simulink model "one_sec_delay_motor_geral_cc"  (R2018b)
settings: Solver=VariableStepAuto  StartTime=0.0  StopTime=10.0  RelTol=1e-3
values from neighbouring files (symbols this model uses):
  b = 0.1    [new_motorCC.m]
  J = 0.01    [new_motorCC.m]
  K = 0.01    [new_motorCC.m]
  L = 0.5    [new_motorCC.m]
  R = 1    [new_motorCC.m]
settings Model: Creator=CarlosHenriqueTorres  LastModifiedBy=CarlosHenriqueTorres

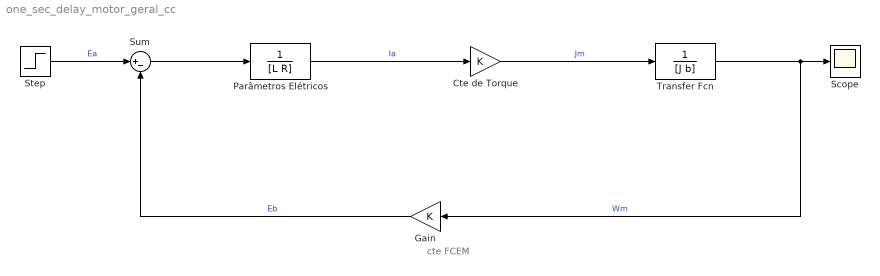
== system one_sec_delay_motor_geral_cc ==
  note: cte FCEM
  Cte de Torque : Gain  Gain=K
  Gain : Gain  Gain=K
  Parâmetros Elétricos : TransferFcn  Denominator=[L R]
  Scope : Scope
  Step : Step  Before=1  SampleTime=0
  Sum : Sum  Inputs=|+-
  Transfer Fcn : TransferFcn  Denominator=[J b]
  wires:
  Parâmetros Elétricos/1 -> Cte de Torque/1  "Ia"
  Transfer Fcn/1 -> Gain/1, Scope/1  "Wm"
  Step/1 -> Sum/1  "Ea"
  Sum/1 -> Parâmetros Elétricos/1
  Gain/1 -> Sum/2  "Eb"
  Cte de Torque/1 -> Transfer Fcn/1  "Jm"
